simulink model "Disparity_CT_old"  (R2021a)
settings: Solver=VariableStepAuto  StartTime=0.0  StopTime=840000  RelTol=1e-3
undefined symbols (not defined in the file or in its folder): imgColSize, imgRowSize
libraries: hdlsllib x9, visionhdlio x2, visionsources x1
settings Model: Creator=user  LastModifiedBy=user
settings OptimizationCC: BlockReduction=off  ConditionallyExecuteInputs=off  DefaultParameterBehavior=Inlined
settings DebuggingCC: AlgebraicLoopMsg=error
settings HardwareCC: ProdBitPerPointer=32  ProdBitPerSizeT=32  ProdBitPerPtrDiffT=32  ProdLargestAtomicFloat=None  ProdIntDivRoundTo=Undefined  ProdEndianess=Unspecified  ProdWordSize=32  ProdHWDeviceType=ASIC/FPGA->ASIC/FPGA  TargetBitPerPointer=64  TargetBitPerSizeT=64  TargetBitPerPtrDiffT=64  TargetLongLongMode=on  TargetIntDivRoundTo=Zero  TargetEndianess=LittleEndian  TargetWordSize=64  TargetHWDeviceType=Custom Processor->MATLAB Host Computer  ProdEqTarget=off

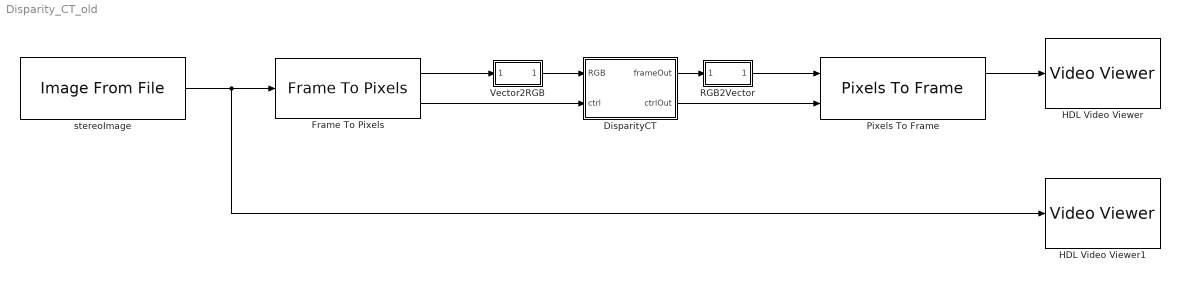
== system Disparity_CT_old ==
  DisparityCT : Subsystem  TreatAsAtomicUnit=on
  Frame To Pixels : visionhdlio/Frame To Pixels  NumComponents=3  NumPixels=1  VideoFormat=480p  ActivePixelsPerLine=imgColSize  ActiveVideoLines=imgRowSize  TotalPixelsPerLine=imgColSize+90  TotalVideoLines=imgRowSize+60  StartingActiveLine=31  FrontPorch=45  SampleTime=0
      settings: SourceProductBaseCode=VT
  HDL Video Viewer : VideoViewer  useColorMap=on  FigPos=[121 747 756 478]
  HDL Video Viewer1 : VideoViewer  useColorMap=on  FigPos=[870 748 756 478]
  Pixels To Frame : visionhdlio/Pixels To Frame  NumComponents=3  NumPixels=1  VideoFormat=480p  ActivePixelsPerLine=imgColSize  ActiveVideoLines=imgRowSize  TotalPixelsPerLine=imgColSize+90  TotalVideoLines=imgRowSize+60
      settings: SourceProductBaseCode=VT
  RGB2Vector : Subsystem
  Vector2RGB : Subsystem
  stereoImage : visionsources/Image From File  Tag=vipblks_nd  FileName=D:\Work\XilFPGAdev\Custom_IP_Cores\SimulinkHDLCoder\SGBMDisparity\stereoTestimg_01_480p.bmp  Ts=420000  imagePorts=One multidimensional signal  OutPortLabels=R|G|B  ImageDataType=Inherit from input image  sdImageDataType=uint(8)  Signed=on  WordLength=16  FractionLengthMode=User-defined  FractionLength=15
  wires:
  RGB2Vector/1(RGBVector) -> Pixels To Frame/1
  DisparityCT/1(frameOut) -> RGB2Vector/1(RGB)
  Vector2RGB/1(RGB) -> DisparityCT/1(RGB)
  Frame To Pixels/2 -> DisparityCT/2(ctrl)
  Pixels To Frame/1 -> HDL Video Viewer/1
  stereoImage/1 -> HDL Video Viewer1/1, Frame To Pixels/1
  Frame To Pixels/1 -> Vector2RGB/1(RGBVector)
  DisparityCT/2(ctrlOut) -> Pixels To Frame/2

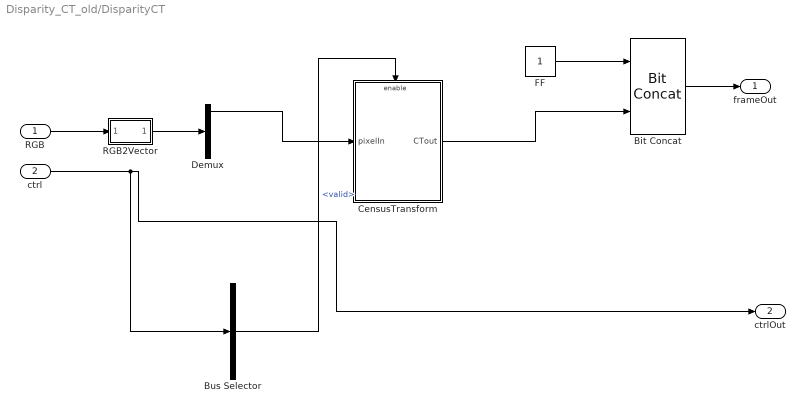
== system Disparity_CT_old/DisparityCT ==
  RGB : Inport
  ctrl : Inport  Port=2
  Bit Concat : hdlsllib/Logic and Bit Operations/Bit Concat  numInputs=2
  Bus Selector : BusSelector  OutputSignals=valid
  CensusTransform : Subsystem
  Demux : Demux  Outputs=3
  FF : Constant  OutDataTypeStr=boolean  SampleTime=-1
  RGB2Vector : Subsystem
  frameOut : Outport
  ctrlOut : Outport  Port=2  VectorParamsAs1DForOutWhenUnconnected=off
  wires:
  RGB/1 -> RGB2Vector/1(RGB)
  RGB2Vector/1(RGBVector) -> Demux/1
  Bit Concat/1 -> frameOut/1
  Demux/1 -> CensusTransform/1(pixelIn)
  FF/1 -> Bit Concat/1
  CensusTransform/1(CTout) -> Bit Concat/2
  Bus Selector/1 -> CensusTransform/Enable  "<valid>"
  ctrl/1 -> ctrlOut/1, Bus Selector/1

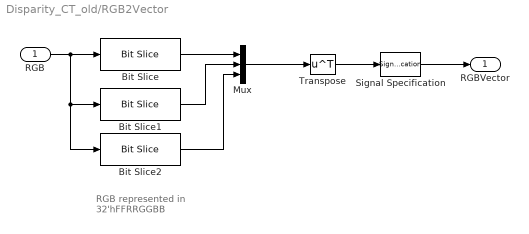
== system Disparity_CT_old/RGB2Vector ==
  note: RGB represented in
      | 32'hFFRRGGBB
  RGB : Inport
  Bit Slice : hdlsllib/Logic and Bit Operations/Bit Slice  lidx=23  ridx=16
      settings: SourceProductBaseCode=SL
  Bit Slice1 : hdlsllib/Logic and Bit Operations/Bit Slice  lidx=15  ridx=8
      settings: SourceProductBaseCode=SL
  Bit Slice2 : hdlsllib/Logic and Bit Operations/Bit Slice  lidx=7  ridx=0
      settings: SourceProductBaseCode=SL
  Mux : Mux  Inputs=3
  Signal Specification : SignalSpecification
  Transpose : Math  Operator=transpose  SignedPower=on  SaturateOnIntegerOverflow=on
  RGBVector : Outport  VectorParamsAs1DForOutWhenUnconnected=off
  wires:
  Mux/1 -> Transpose/1
  Bit Slice/1 -> Mux/1
  Bit Slice2/1 -> Mux/3
  Bit Slice1/1 -> Mux/2
  RGB/1 -> Bit Slice2/1, Bit Slice1/1, Bit Slice/1
  Transpose/1 -> Signal Specification/1
  Signal Specification/1 -> RGBVector/1

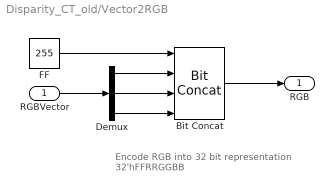
== system Disparity_CT_old/Vector2RGB ==
  note: Encode RGB into 32 bit representation
      | 32'hFFRRGGBB
  RGBVector : Inport
  Bit Concat : hdlsllib/Logic and Bit Operations/Bit Concat  numInputs=4
  Demux : Demux  Outputs=3
  FF : Constant  Value=255  OutDataTypeStr=uint8  SampleTime=-1
  RGB : Outport  VectorParamsAs1DForOutWhenUnconnected=off
  wires:
  Bit Concat/1 -> RGB/1
  RGBVector/1 -> Demux/1
  FF/1 -> Bit Concat/1
  Demux/1 -> Bit Concat/2
  Demux/2 -> Bit Concat/3
  Demux/3 -> Bit Concat/4

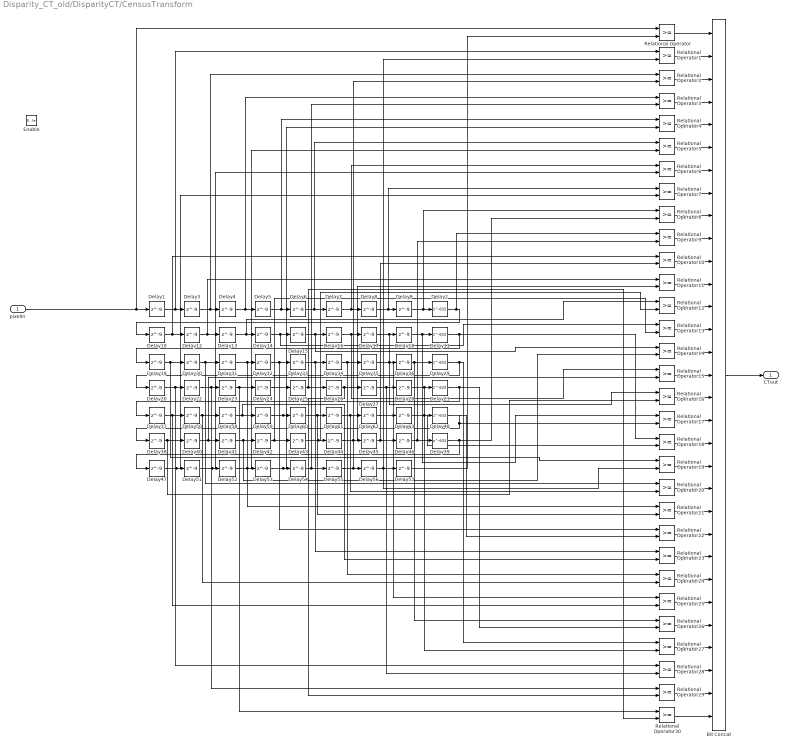
== system Disparity_CT_old/DisparityCT/CensusTransform ==
  pixelIn : Inport
  Enable : EnablePort
  Bit Concat : hdlsllib/Logic and Bit Operations/Bit Concat  numInputs=31
  Delay{1,3..10,12..20,22..28,30..38,40..47,50..63} (56 alike) : Delay  DelayLength=9
  Delay{2,11,21,29,39,48} (6 alike) : Delay  DelayLength=632
  Relational Operator{,1..30} (31 alike) : RelationalOperator  OutDataTypeStr=boolean  RndMeth=Nearest
  CTout : Outport  InitialOutput=0  VectorParamsAs1DForOutWhenUnconnected=off
  wires:
  pixelIn/1 -> Relational Operator/1, Delay1/1
  Bit Concat/1 -> CTout/1
  Delay1/1 -> Relational Operator1/1, Delay3/1
  Delay3/1 -> Relational Operator2/1, Delay4/1
  Delay4/1 -> Relational Operator3/1, Delay5/1
  Delay5/1 -> Relational Operator4/1, Delay6/1
  Delay6/1 -> Relational Operator5/1, Delay7/1
  Delay7/1 -> Relational Operator6/1, Delay8/1
  Delay8/1 -> Relational Operator7/1, Delay9/1
  Delay9/1 -> Relational Operator8/1, Delay2/1
  Delay16/1 -> Relational Operator15/1, Delay17/1
  Delay18/1 -> Relational Operator17/1, Delay11/1
  Delay13/1 -> Relational Operator12/1, Delay14/1
  Delay15/1 -> Relational Operator14/1, Delay16/1
  Delay10/1 -> Relational Operator10/1, Delay12/1
  Delay12/1 -> Relational Operator11/1, Delay13/1
  Delay17/1 -> Relational Operator16/1, Delay18/1
  Delay14/1 -> Relational Operator13/1, Delay15/1
  Delay34/1 -> Relational Operator24/1, Delay35/1
  Delay31/1 -> Relational Operator21/1, Delay32/1
  Delay36/1 -> Relational Operator26/1, Delay29/1
  Delay27/1 -> Relational Operator28/2, Delay28/1
  Delay25/1 -> Delay26/1, Relational Operator30/2
  Delay20/1 -> Relational Operator28/1, Delay22/1
  Delay26/1 -> Relational Operator29/2, Delay27/1
  Delay23/1 -> Relational Operator30/1, Delay24/1
  Delay33/1 -> Relational Operator23/1, Delay34/1
  Delay19/1 -> Relational Operator19/1, Delay30/1
  Delay24/1 -> Delay25/1
  Delay30/1 -> Relational Operator20/1, Delay31/1
  Delay35/1 -> Relational Operator25/1, Delay36/1
  Delay32/1 -> Relational Operator22/1, Delay33/1
  Delay28/1 -> Relational Operator27/2, Delay21/1
  Delay22/1 -> Relational Operator29/1, Delay23/1
  Delay61/1 -> Relational Operator20/2, Delay62/1
  Delay58/1 -> Relational Operator23/2, Delay59/1
  Delay63/1 -> Relational Operator18/2, Delay48/1
  Delay43/1 -> Relational Operator12/2, Delay44/1
  Delay38/1 -> Delay40/1, Relational Operator16/2
  Delay41/1 -> Relational Operator14/2, Delay42/1
  Delay60/1 -> Relational Operator21/2, Delay61/1
  Delay37/1 -> Relational Operator25/2, Delay50/1
  Delay42/1 -> Relational Operator13/2, Delay43/1
  Delay50/1 -> Relational Operator24/2, Delay58/1
  Delay62/1 -> Delay63/1
  Delay47/1 -> Relational Operator7/2, Delay51/1
  Delay56/1 -> Relational Operator1/2, Relational Operator19/2, Delay57/1
  Delay54/1 -> Relational Operator3/2, Delay55/1
  Delay45/1 -> Delay46/1, Relational Operator10/2
  Delay51/1 -> Relational Operator6/2, Delay52/1
  Delay44/1 -> Relational Operator11/2, Delay45/1
  Delay53/1 -> Relational Operator4/2, Delay54/1
  Delay55/1 -> Relational Operator2/2, Delay56/1
  Delay59/1 -> Relational Operator22/2, Delay60/1
  Delay46/1 -> Relational Operator9/2, Delay39/1
  Delay40/1 -> Relational Operator15/2, Delay41/1
  Delay52/1 -> Relational Operator5/2, Delay53/1
  Delay2/1 -> Relational Operator9/1, Delay10/1
  Delay11/1 -> Relational Operator18/1, Delay19/1
  Delay29/1 -> Relational Operator27/1, Delay20/1
  Delay21/1 -> Relational Operator26/2, Delay37/1
  Delay48/1 -> Relational Operator17/2, Delay38/1
  Delay39/1 -> Relational Operator8/2, Delay47/1
  Relational Operator/1 -> Bit Concat/1
  Relational Operator1/1 -> Bit Concat/2
  Relational Operator2/1 -> Bit Concat/3
  Relational Operator3/1 -> Bit Concat/4
  Relational Operator4/1 -> Bit Concat/5
  Relational Operator7/1 -> Bit Concat/8
  Relational Operator5/1 -> Bit Concat/6
  Relational Operator6/1 -> Bit Concat/7
  Relational Operator14/1 -> Bit Concat/15
  Relational Operator12/1 -> Bit Concat/13
  Relational Operator15/1 -> Bit Concat/16
  Relational Operator13/1 -> Bit Concat/14
  Relational Operator8/1 -> Bit Concat/9
  Relational Operator11/1 -> Bit Concat/12
  Relational Operator9/1 -> Bit Concat/10
  Relational Operator10/1 -> Bit Concat/11
  Relational Operator22/1 -> Bit Concat/23
  Relational Operator20/1 -> Bit Concat/21
  Relational Operator23/1 -> Bit Concat/24
  Relational Operator21/1 -> Bit Concat/22
  Relational Operator16/1 -> Bit Concat/17
  Relational Operator19/1 -> Bit Concat/20
  Relational Operator17/1 -> Bit Concat/18
  Relational Operator18/1 -> Bit Concat/19
  Relational Operator30/1 -> Bit Concat/31
  Relational Operator28/1 -> Bit Concat/29
  Relational Operator29/1 -> Bit Concat/30
  Relational Operator24/1 -> Bit Concat/25
  Relational Operator27/1 -> Bit Concat/28
  Relational Operator25/1 -> Bit Concat/26
  Relational Operator26/1 -> Bit Concat/27
  Delay57/1 -> Relational Operator/2

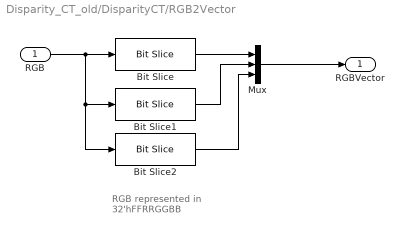
== system Disparity_CT_old/DisparityCT/RGB2Vector ==
  note: RGB represented in
      | 32'hFFRRGGBB
  RGB : Inport
  Bit Slice : hdlsllib/Logic and Bit Operations/Bit Slice  lidx=23  ridx=16
      settings: SourceProductBaseCode=SL
  Bit Slice1 : hdlsllib/Logic and Bit Operations/Bit Slice  lidx=15  ridx=8
      settings: SourceProductBaseCode=SL
  Bit Slice2 : hdlsllib/Logic and Bit Operations/Bit Slice  lidx=7  ridx=0
      settings: SourceProductBaseCode=SL
  Mux : Mux  Inputs=3
  RGBVector : Outport  VectorParamsAs1DForOutWhenUnconnected=off
  wires:
  Bit Slice/1 -> Mux/1
  Bit Slice2/1 -> Mux/3
  Bit Slice1/1 -> Mux/2
  RGB/1 -> Bit Slice2/1, Bit Slice1/1, Bit Slice/1
  Mux/1 -> RGBVector/1
